simulink model "TP_Moteur_BO"  (R2012b)
settings: Solver=ode4  StartTime=0.0  StopTime=9999  FixedStep=Te  RelTol=1e-3
undefined symbols (not defined in the file): EE2, K, National_Instruments, obsver, P, PCI, tau_i, Te
libraries: rtwinlib x2
settings Model: SimulationMode=external  Creator=sylvain  LastModifiedBy=m2istr_13
settings DataIOCC: MaxDataPoints=5000  SignalLoggingSaveFormat=ModelDataLogs
settings OptimizationCC: BlockReduction=off  BooleanDataType=off  InlineInvariantSignals=on
settings DebuggingCC: SaveWithParameterizedLinksMsg=none  SignalResolutionControl=TryResolveAllWithWarning  SolverPrmCheckMsg=none  MultiTaskDSMMsg=warning  MultiTaskCondExecSysMsg=none  StrictBusMsg=None
settings HardwareCC: ProdIntDivRoundTo=Zero  ProdEndianess=LittleEndian  ProdHWDeviceType=Generic->32-bit x86 compatible  TargetIntDivRoundTo=Zero  TargetEndianess=LittleEndian  TargetHWDeviceType=MATLAB Host  ProdEqTarget=off
settings RTWCC: SystemTargetFile=rtwin.tlc  TemplateMakefile=rtwin.tmf  Description=Real-Time Windows Target  ProcessScript=rtwin_make_rtw_hook  IncludeERTFirstTime=on  RTWCompilerOptimization=On
settings CodeAppCC: MaxIdLength=95
settings RTWinTargetCC: TargetLibSuffix=_rtwin.lib  TargetPreCompLibLocation=C:\Program Files\MATLAB\R2012b\toolbox\rtw\targets\rtwin\lib\win32  CodeReplacementLibrary=ANSI_C  RTWinDir=C:/PROGRA~1/MATLAB/R2012b/toolbox/rtw/targets/rtwin  TargetArch=win32

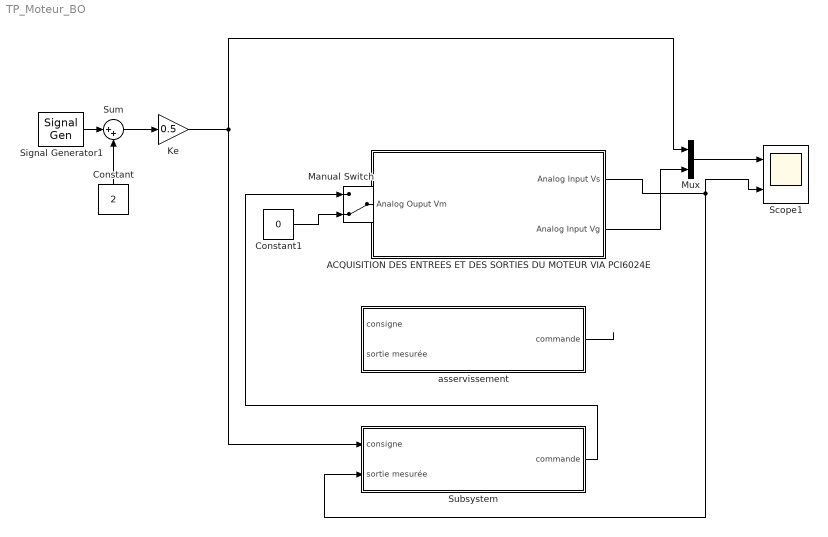
== system TP_Moteur_BO ==
  ACQUISITION DES ENTREES ET DES SORTIES DU MOTEUR VIA PCI6024E : Subsystem
  Constant : Constant  Value=2
  Constant1 : Constant  Value=0
  Ke : Gain  Gain=0.5  SaturateOnIntegerOverflow=on  OutDataTypeStr=Inherit: Same as input  ParamDataTypeStr=Inherit: Same as input
  Manual Switch : ManualSwitch  CurrentSetting=0
  Mux : Mux  Inputs=2
  Scope1 : Scope  NumInputPorts=2
      settings: TimeRange=3  YMin=-5.5~-5.5  YMax=5.5~5.5  SaveName=y  DataFormat=Structure
  Signal Generator1 : SignalGenerator  WaveForm=square  Amplitude=2  Frequency=0.1
  Subsystem : Subsystem
  Sum : Sum  Inputs=|++  SaturateOnIntegerOverflow=on  InputSameDT=on  OutDataTypeStr=Inherit: Same as first input
  asservissement : Subsystem
  wires:
  Ke/1 -> Subsystem/1(consigne), Mux/1
  Sum/1 -> Ke/1
  Signal Generator1/1 -> Sum/1
  Constant/1 -> Sum/2
  Mux/1 -> Scope1/1
  Manual Switch/1 -> ACQUISITION DES ENTREES ET DES SORTIES DU MOTEUR VIA PCI6024E/1(Analog Ouput Vm)
  Constant1/1 -> Manual Switch/2
  ACQUISITION DES ENTREES ET DES SORTIES DU MOTEUR VIA PCI6024E/2(Analog Input Vg) -> Mux/2
  ACQUISITION DES ENTREES ET DES SORTIES DU MOTEUR VIA PCI6024E/1(Analog Input Vs) -> Subsystem/2(sortie mesurée), Scope1/2
  asservissement/1(commande) -> ?
  Subsystem/1(commande) -> Manual Switch/1

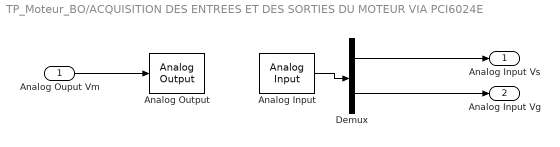
== system TP_Moteur_BO/ACQUISITION DES ENTREES ET DES SORTIES DU MOTEUR VIA PCI6024E ==
  Analog Ouput Vm : Inport
  Analog Input : rtwinlib/Analog Input  SampleTime=Te  MaxMissedTicks=10  ShowMissedTicks=off  YieldWhenWaiting=off  DrvName=National_Instruments/PCI-6024E  DrvAddress=0  DrvOptions=[0 0 0 0 0 0]  Channels=[1 2]  RangeMode=1  VoltRange=1  DataType=1
      settings: AttributesFormatString=National Instruments\nPCI-6024E [0h]
  Analog Output : rtwinlib/Analog Output  SampleTime=Te  MaxMissedTicks=10  ShowMissedTicks=off  YieldWhenWaiting=off  DrvName=National_Instruments/PCI-6024E  DrvAddress=0  DrvOptions=[0 0 0 0 0 0]  Channels=1  RangeMode=1  VoltRange=1  InitialValue=[]  FinalValue=[]
      settings: AttributesFormatString=National Instruments\nPCI-6024E [0h]
  Demux : Demux  Outputs=2
  Analog Input Vs : Outport
  Analog Input Vg : Outport  Port=2
  wires:
  Analog Input/1 -> Demux/1
  Demux/2 -> Analog Input Vg/1
  Analog Ouput Vm/1 -> Analog Output/1
  Demux/1 -> Analog Input Vs/1

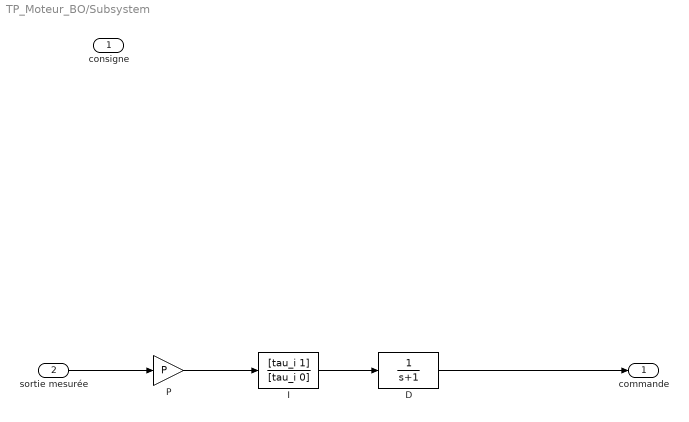
== system TP_Moteur_BO/Subsystem ==
  consigne : Inport
  sortie mesurée : Inport  Port=2
  D : TransferFcn  Denominator=[1 1]
  I : TransferFcn  Numerator=[tau_i 1]  Denominator=[tau_i 0]
  P : Gain  Gain=P
  commande : Outport
  wires:
  I/1 -> D/1
  D/1 -> commande/1
  P/1 -> I/1
  sortie mesurée/1 -> P/1

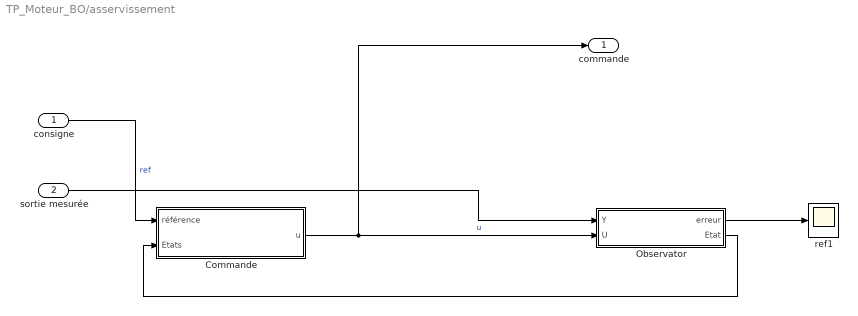
== system TP_Moteur_BO/asservissement ==
  consigne : Inport
  sortie mesurée : Inport  Port=2
  "Commande " : Subsystem
  Observator : Subsystem
  ref1 : Scope
      settings: SaveName=ScopeData4
  commande : Outport
  wires:
  consigne/1 -> "Commande "/1(référence)  "ref"
  Observator/2("Etat ") -> "Commande "/2(Etats)
  sortie mesurée/1 -> Observator/1("Y ")
  "Commande "/1(u) -> Observator/2(U), commande/1  "u"
  Observator/1(erreur) -> ref1/1

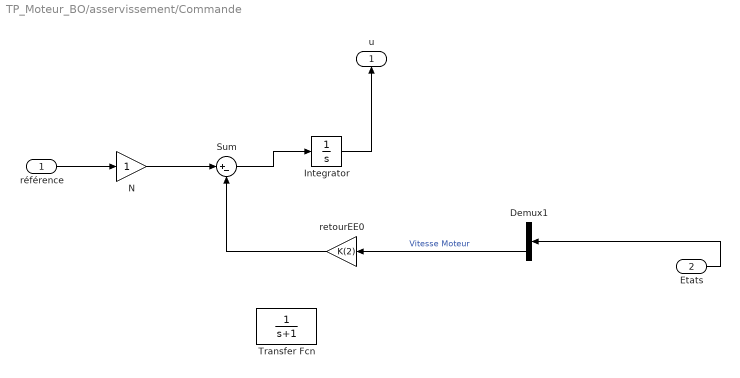
== system TP_Moteur_BO/asservissement/Commande  ==
  référence : Inport
  Etats : Inport  Port=2
  Demux1 : Demux  Outputs=2
  Integrator : Integrator
  "N " : Gain
  Sum : Sum  Inputs=|+-
  Transfer Fcn : TransferFcn  Denominator=[1 1]
  retourEE0 : Gain  Gain=K(2)
  u : Outport
  wires:
  Sum/1 -> Integrator/1
  référence/1 -> "N "/1
  Etats/1 -> Demux1/1
  retourEE0/1 -> Sum/2
  "N "/1 -> Sum/1
  Demux1/2 -> retourEE0/1  "Vitesse Moteur"
  Integrator/1 -> u/1

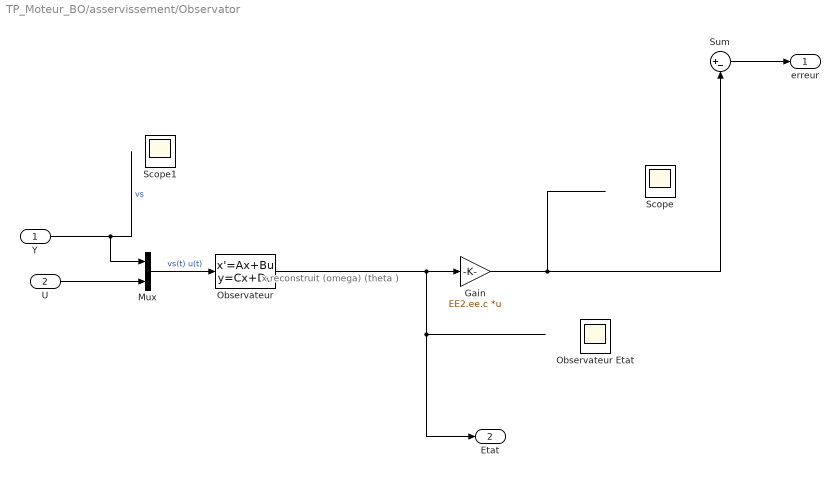
== system TP_Moteur_BO/asservissement/Observator ==
  note: x reconstruit
      | (omega)
      | (theta   )
  "Y " : Inport
  U : Inport  Port=2
  Gain : Gain  Gain=EE2.ee.c  Multiplication=Matrix(K*u)
  Mux : Mux  Inputs=2
  "Observateur " : StateSpace  A=obsver.ee.a  B=obsver.ee.b  C=obsver.ee.c  D=obsver.ee.d
  "Observateur Etat " : Scope
  Scope : Scope
      settings: YMin=-600  YMax=600
  Scope1 : Scope
      settings: YMin=16  YMax=30  SaveName=ScopeData2
  Sum : Sum  Inputs=|+-
  erreur : Outport
  "Etat " : Outport  Port=2
  wires:
  "Observateur "/1 -> "Etat "/1, Gain/1
  "Y "/1 -> Mux/1  "vs"
  Sum/1 -> erreur/1
  Mux/1 -> "Observateur "/1  "vs(t) u(t)"
  Gain/1 -> Sum/2
  U/1 -> Mux/2
